simulink model "HANcoder_E407_SMV_program"  (R2018a)
settings: Solver=FixedStepDiscrete  StartTime=0.0  StopTime=1  FixedStep=0.01  RelTol=1e-3
PreLoadFcn:
  | librarySetup
  | eval([bdroot,'_startup']) %Calling [modelName]_startup.m
values from neighbouring files (symbols this model uses):
  Speed = [0.4; 0.4; 0.4; 0.4; 0.4; 0.4; 0.4; 0.4; 0.4; 0.4;0]    [Xbee_Track_Presentation.m]
undefined symbols (not defined in the file or in its folder): A0, A1, A2, A3, b, CON2, CON3, CON4, D13, D4, D5, drivemode, L_D1, L_D2, manual_xbee_switch, Steering_angle, steermode
libraries: HANcoder_STM32_Target x38, simulink_extras x11, simulink x7
(part 2 of 3)

== system HANcoder_E407_SMV_program/HANcoder STM32 Target - E407-STM32 algorithm/Xbee controll/Error value als het nodig is ==
  ThrottleIn : Inport
  SteeringIn : Inport  Port=2
  SteeringOut : Outport
  ThrottleOut : Outport  Port=2
  wires:
  ThrottleIn/1 -> ThrottleOut/1
  SteeringIn/1 -> SteeringOut/1

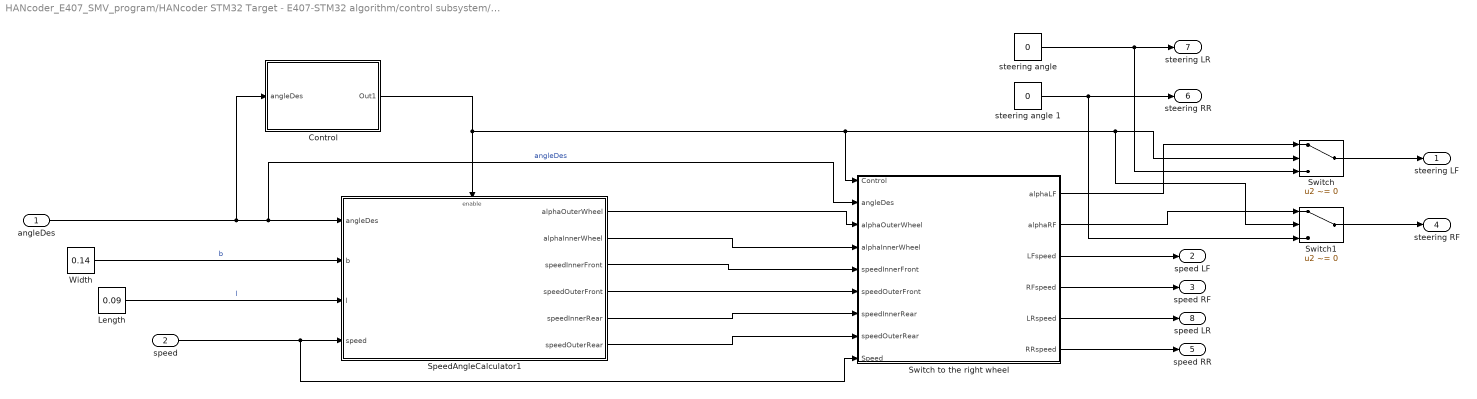
== system HANcoder_E407_SMV_program/HANcoder STM32 Target - E407-STM32 algorithm/control subsystem/2 wheel steering ==
  angleDes : Inport
  speed : Inport  Port=2
  Control : Subsystem
  Length : Constant  Value=0.09
  SpeedAngleCalculator1 : Subsystem
  Switch : Switch  Criteria=u2 ~= 0
  "Switch to the right wheel " : Subsystem
  Switch1 : Switch  Criteria=u2 ~= 0
  Width : Constant  Value=0.14
  "steering angle " : Constant  Value=0
  steering angle 1 : Constant  Value=0
  steering LF : Outport
  speed LF : Outport  Port=2
  speed RF : Outport  Port=3
  steering RF : Outport  Port=4
  speed RR : Outport  Port=5
  steering RR : Outport  Port=6
  steering LR : Outport  Port=7
  speed LR : Outport  Port=8
  wires:
  "steering angle "/1 -> Switch/3, steering LR/1
  steering angle 1/1 -> Switch1/3, steering RR/1
  "Switch to the right wheel "/4(RFspeed) -> speed RF/1
  angleDes/1 -> Control/1(angleDes), "Switch to the right wheel "/2(angleDes), SpeedAngleCalculator1/1(angleDes)  "angleDes"
  "Switch to the right wheel "/5(LRspeed) -> speed LR/1
  "Switch to the right wheel "/6(RRspeed) -> speed RR/1
  speed/1 -> "Switch to the right wheel "/9(Speed), SpeedAngleCalculator1/4(speed)
  Width/1 -> SpeedAngleCalculator1/2(b)  "b"
  SpeedAngleCalculator1/2(alphaInnerWheel) -> "Switch to the right wheel "/4(alphaInnerWheel)
  SpeedAngleCalculator1/6(speedOuterRear) -> "Switch to the right wheel "/8(speedOuterRear)
  SpeedAngleCalculator1/5(speedInnerRear) -> "Switch to the right wheel "/7(speedInnerRear)
  Length/1 -> SpeedAngleCalculator1/3(l)  "l"
  SpeedAngleCalculator1/1(alphaOuterWheel) -> "Switch to the right wheel "/3(alphaOuterWheel)
  SpeedAngleCalculator1/3(speedInnerFront) -> "Switch to the right wheel "/5(speedInnerFront)
  "Switch to the right wheel "/3(LFspeed) -> speed LF/1
  SpeedAngleCalculator1/4(speedOuterFront) -> "Switch to the right wheel "/6(speedOuterFront)
  "Switch to the right wheel "/1(alphaLF) -> Switch/1
  Switch/1 -> steering LF/1
  Switch1/1 -> steering RF/1
  "Switch to the right wheel "/2(alphaRF) -> Switch1/1
  Control/1(Out1) -> "Switch to the right wheel "/1(Control), Switch1/2, Switch/2, SpeedAngleCalculator1/Enable

== system HANcoder_E407_SMV_program/HANcoder STM32 Target - E407-STM32 algorithm/control subsystem/4 wheel steering ==
  angleDes : Inport
  speed : Inport  Port=2
  Control : Subsystem
  Subsystem1 : Subsystem
  Switch to the right wheel (Don't open if you're smart)1 : Subsystem
  angleDes1 : InportShadow
  angleDes2 : InportShadow
  b : Constant  Value=0.14
  l : Constant  Value=0.09
  speed2 : InportShadow  Port=2
  steering LF : Outport
  speed LF : Outport  Port=2
  speed RF : Outport  Port=3
  steering RF : Outport  Port=4
  speed RR : Outport  Port=5
  steering RR : Outport  Port=6
  steering LR : Outport  Port=7
  speed LR : Outport  Port=8
  wires:
  Switch to the right wheel (Don't open if you're smart)1/5(LFspeed) -> speed LF/1
  Switch to the right wheel (Don't open if you're smart)1/4(steeringRR) -> steering RR/1
  Switch to the right wheel (Don't open if you're smart)1/8(RRspeed) -> speed RR/1
  Switch to the right wheel (Don't open if you're smart)1/3(steeringRF) -> steering RF/1
  Switch to the right wheel (Don't open if you're smart)1/2("steeringLR ") -> steering LR/1
  Switch to the right wheel (Don't open if you're smart)1/6(RFspeed) -> speed RF/1
  Switch to the right wheel (Don't open if you're smart)1/7(LRspeed) -> speed LR/1
  Switch to the right wheel (Don't open if you're smart)1/1(steeringLF) -> steering LF/1
  angleDes2/1 -> Switch to the right wheel (Don't open if you're smart)1/6(angleDes)
  speed/1 -> Switch to the right wheel (Don't open if you're smart)1/7(Speed)
  b/1 -> Subsystem1/3(b)
  Subsystem1/2(speedOuter) -> Switch to the right wheel (Don't open if you're smart)1/3(speedOuterFront)
  l/1 -> Subsystem1/1(l)
  Subsystem1/4(AlphaInner) -> Switch to the right wheel (Don't open if you're smart)1/5(alphaOuterWheel)
  Control/1(Control) -> Subsystem1/Enable, Switch to the right wheel (Don't open if you're smart)1/1(Control)
  Subsystem1/3(AlphaOuter) -> Switch to the right wheel (Don't open if you're smart)1/4(alphaInnerWheel)
  Subsystem1/1(speedInner) -> Switch to the right wheel (Don't open if you're smart)1/2(speedInnerFront)
  angleDes/1 -> Subsystem1/2(angleDes)
  angleDes1/1 -> Control/1(angleDes)
  speed2/1 -> Subsystem1/4(speed)

== system HANcoder_E407_SMV_program/HANcoder STM32 Target - E407-STM32 algorithm/control subsystem/axle enable ==
  Xbeedriveline : Inport
  incomingF : Inport  Port=2
  incomingR : Inport  Port=3
  Subsystem : Subsystem
  Subsystem1 : Subsystem
  Out1 : Outport
  Out2 : Outport  Port=2
  wires:
  Subsystem/1(zero1) -> Out2/1
  Subsystem1/1(zero) -> Out1/1
  Xbeedriveline/1 -> Subsystem/2(xbeedriveline), Subsystem1/2(xbeedriveline)
  incomingF/1 -> Subsystem1/1(incomingF)
  incomingR/1 -> Subsystem/1(incomingR)

== system HANcoder_E407_SMV_program/HANcoder STM32 Target - E407-STM32 algorithm/control subsystem/direction subsystem ==
  Xbeedrive : Inport
  Constant : Constant  Value=3
  Digital Output1 : HANcoder_STM32_Target/STM32-E407/Digital Outputs/Digital Output  Tag=HANcoder_TARGET_STM32_E407  pinID=CON PE - 4  config=Push pull  tsamp=-1
      settings: SourceProductName=HANcoder STM32 Target
  Sum : Sum  Inputs=|+-
  Switch : Switch  Threshold=4  OutDataTypeStr=boolean
  Switch1 : Switch  Threshold=1
  negDirection : Constant
  posDirection : Constant  Value=0
  Out1 : Outport
  wires:
  negDirection/1 -> Switch/1
  Xbeedrive/1 -> Switch1/3, Sum/1, Switch/2
  Switch/1 -> Switch1/2, Digital Output1/1  "direction"
  posDirection/1 -> Switch/3
  Constant/1 -> Sum/2
  Switch1/1 -> Out1/1
  Sum/1 -> Switch1/1

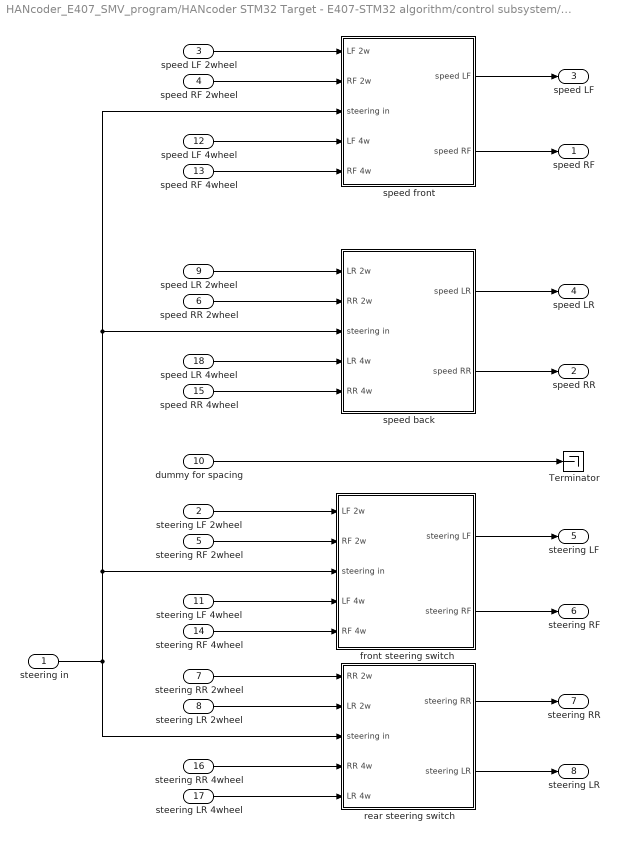
== system HANcoder_E407_SMV_program/HANcoder STM32 Target - E407-STM32 algorithm/control subsystem/steering switch ==
  steering in : Inport
  steering LF 2wheel : Inport  Port=2
  speed LF 2wheel : Inport  Port=3
  speed RF 2wheel : Inport  Port=4
  steering RF 2wheel : Inport  Port=5
  speed RR 2wheel : Inport  Port=6
  steering RR 2wheel : Inport  Port=7
  steering LR 2wheel : Inport  Port=8
  speed LR 2wheel : Inport  Port=9
  dummy for spacing : Inport  Port=10
  steering LF 4wheel : Inport  Port=11
  speed LF 4wheel : Inport  Port=12
  speed RF 4wheel : Inport  Port=13
  steering RF 4wheel : Inport  Port=14
  speed RR 4wheel : Inport  Port=15
  steering RR 4wheel : Inport  Port=16
  steering LR 4wheel : Inport  Port=17
  speed LR 4wheel : Inport  Port=18
  Terminator : Terminator
  front steering switch : Subsystem
  rear steering switch : Subsystem
  speed back : Subsystem
  speed front : Subsystem
  speed RF : Outport
  speed RR : Outport  Port=2
  speed LF : Outport  Port=3
  speed LR : Outport  Port=4
  steering LF : Outport  Port=5
  steering RF : Outport  Port=6
  steering RR : Outport  Port=7
  steering LR : Outport  Port=8
  wires:
  rear steering switch/1(steering RR) -> steering RR/1
  rear steering switch/2(steering LR) -> steering LR/1
  steering in/1 -> rear steering switch/3(steering in), speed front/3(steering in), speed back/3(steering in), front steering switch/3(steering in)
  speed LR 2wheel/1 -> speed back/1(LR 2w)
  speed LF 2wheel/1 -> speed front/1(LF 2w)
  speed LR 4wheel/1 -> speed back/4(LR 4w)
  speed RR 4wheel/1 -> speed back/5(RR 4w)
  speed RF 2wheel/1 -> speed front/2(RF 2w)
  speed RR 2wheel/1 -> speed back/2(RR 2w)
  front steering switch/2(steering RF) -> steering RF/1
  front steering switch/1(steering LF) -> steering LF/1
  speed LF 4wheel/1 -> speed front/4(LF 4w)
  speed RF 4wheel/1 -> speed front/5(RF 4w)
  steering LF 2wheel/1 -> front steering switch/1(LF 2w)
  steering RF 2wheel/1 -> front steering switch/2(RF 2w)
  steering LF 4wheel/1 -> front steering switch/4(LF 4w)
  steering RF 4wheel/1 -> front steering switch/5(RF 4w)
  steering RR 2wheel/1 -> rear steering switch/1(RR 2w)
  steering LR 2wheel/1 -> rear steering switch/2(LR 2w)
  steering RR 4wheel/1 -> rear steering switch/4(RR 4w)
  steering LR 4wheel/1 -> rear steering switch/5(LR 4w)
  speed front/1(speed LF) -> speed LF/1
  speed front/2(speed RF) -> speed RF/1
  speed back/1(speed LR) -> speed LR/1
  speed back/2(speed RR) -> speed RR/1
  dummy for spacing/1 -> Terminator/1

== system HANcoder_E407_SMV_program/HANcoder STM32 Target - E407-STM32 algorithm/initialisation/Output Compare Init1 ==
  S-Function : S-Function  FunctionName=sfcn_timeout_init  SFunctionDeploymentMode=off  EnableBusSupport=off
  Term1 : Terminator
  wires:
  S-Function/1 -> Term1/1

== system HANcoder_E407_SMV_program/HANcoder STM32 Target - E407-STM32 algorithm/initialisation/PWM Init ==
  S-Function : S-Function  FunctionName=sfcn_pwmout_init  SFunctionDeploymentMode=off  EnableBusSupport=off
  Term1 : Terminator
  wires:
  S-Function/1 -> Term1/1

== system HANcoder_E407_SMV_program/HANcoder STM32 Target - E407-STM32 algorithm/initialisation/PWM Init1 ==
  S-Function : S-Function  FunctionName=sfcn_pwmout_init  SFunctionDeploymentMode=off  EnableBusSupport=off
  Term1 : Terminator
  wires:
  S-Function/1 -> Term1/1

== system HANcoder_E407_SMV_program/HANcoder STM32 Target - E407-STM32 algorithm/initialisation/PWM Init2 ==
  S-Function : S-Function  FunctionName=sfcn_pwmout_init  SFunctionDeploymentMode=off  EnableBusSupport=off
  Term1 : Terminator
  wires:
  S-Function/1 -> Term1/1

== system HANcoder_E407_SMV_program/HANcoder STM32 Target - E407-STM32 algorithm/initialisation/UART init ==
  Level-2 M-file S-Function : M-S-Function  FunctionName=sfcn_uart_init
  Term1 : Terminator
  wires:
  Level-2 M-file S-Function/1 -> Term1/1

== system HANcoder_E407_SMV_program/HANcoder STM32 Target - E407-STM32 algorithm/output compare Left front/Subsystem2 ==
  In1 : Inport
  function : TriggerPort  TriggerType=function-call  VariantControl=(inherit)
  " 2: invert logic state of the outpin pin." : Constant  Value=2  OutDataTypeStr=uint8
  Gain : Gain  Commented=on  Gain=2  OutDataTypeStr=uint16
  Get Free Running Counter1 : HANcoder_STM32_Target/STM32-E407/Timer Outputs/Get Free Running Counter  Tag=HANcoder_TARGET_STM32_E407  moduleID=TIM1 - CON PE - 12 & 14 & 16 & 17  tsamp=-1
      settings: SourceProductName=HANcoder STM32 Target
  Schedule Compare Event1 : HANcoder_STM32_Target/STM32-E407/Timer Outputs/Schedule Compare Event  Tag=HANcoder_TARGET_STM32_E407  pin=TIM1 - CON PE - 12 - 5V Tolerant  tsamp=-1
      settings: SourceProductName=HANcoder STM32 Target
  Sum : Sum  Inputs=|++
  wires:
  " 2: invert logic state of the outpin pin."/1 -> Schedule Compare Event1/2
  Get Free Running Counter1/1 -> Sum/2
  Sum/1 -> Schedule Compare Event1/1
  In1/1 -> Sum/1

== system HANcoder_E407_SMV_program/HANcoder STM32 Target - E407-STM32 algorithm/output compare Left front/calculated frequency ==
  ticks : Inport
  Constant : Constant  Value=10000000  OutDataTypeStr=uint32
  Divide : Product  Inputs=*/  OutDataTypeStr=uint32
  Gain : Gain  Gain=2  OutDataTypeStr=uint16
  Product : Product
  Terminator : Terminator
  t_tick times 10^7 : Constant  Value=5  OutDataTypeStr=uint8
  wires:
  Constant/1 -> Divide/1
  Product/1 -> Divide/2
  Gain/1 -> Product/1
  t_tick times 10^7/1 -> Product/2
  Divide/1 -> Terminator/1  "freq_calc_LF"
  ticks/1 -> Gain/1

== system HANcoder_E407_SMV_program/HANcoder STM32 Target - E407-STM32 algorithm/output compare Left front/ms to tick conversion ==
  note: rad/s
  m/s : Inport
  Constant2 : Constant
  Divide1 : Product  Inputs=*/  OutDataTypeStr=uint16
  Gain : Gain  Gain=2
  Gain1 : Gain  Gain=0.0000005
  Gain2 : Gain  Gain=2*pi
  Gain3 : Gain  Gain=200
  wheel radius : Gain  Gain=1/0.0405
  Out1 : Outport
  wires:
  Constant2/1 -> Gain2/1
  Gain/1 -> Gain1/1
  m/s/1 -> wheel radius/1
  Gain1/1 -> Gain3/1
  Divide1/1 -> Out1/1
  Gain2/1 -> Divide1/1
  Gain3/1 -> Divide1/2
  wheel radius/1 -> Gain/1

== system HANcoder_E407_SMV_program/HANcoder STM32 Target - E407-STM32 algorithm/output compare Left front/start scheduling for output compare ==
  Trigger : TriggerPort  TriggerType=either  VariantControl=(inherit)  InitialTriggerSignalState=zero  PortDimensions=1
  "  3: do nothing to the output pin." : Constant  Value=3  OutDataTypeStr=uint8
  Schedule Compare Event : HANcoder_STM32_Target/STM32-E407/Timer Outputs/Schedule Compare Event  Tag=HANcoder_TARGET_STM32_E407  pin=TIM1 - CON PE - 12 - 5V Tolerant  tsamp=-1
      settings: SourceProductName=HANcoder STM32 Target
  zero value : Constant  Value=0  OutDataTypeStr=uint16
  wires:
  "  3: do nothing to the output pin."/1 -> Schedule Compare Event/2
  zero value/1 -> Schedule Compare Event/1

== system HANcoder_E407_SMV_program/HANcoder STM32 Target - E407-STM32 algorithm/output compare left rear/Subsystem2 ==
  In1 : Inport
  function : TriggerPort  TriggerType=function-call  VariantControl=(inherit)
  " 2: invert logic state of the outpin pin." : Constant  Value=2  OutDataTypeStr=uint8
  Get Free Running Counter1 : HANcoder_STM32_Target/STM32-E407/Timer Outputs/Get Free Running Counter  Tag=HANcoder_TARGET_STM32_E407  moduleID=TIM1 - CON PE - 12 & 14 & 16 & 17  tsamp=-1
      settings: SourceProductName=HANcoder STM32 Target
  Schedule Compare Event1 : HANcoder_STM32_Target/STM32-E407/Timer Outputs/Schedule Compare Event  Tag=HANcoder_TARGET_STM32_E407  pin=TIM1 - CON PE - 17 - 5V Tolerant  tsamp=-1
      settings: SourceProductName=HANcoder STM32 Target
  Sum : Sum  Inputs=|++  OutDataTypeStr=uint16
  wires:
  Sum/1 -> Schedule Compare Event1/1
  Get Free Running Counter1/1 -> Sum/2
  " 2: invert logic state of the outpin pin."/1 -> Schedule Compare Event1/2
  In1/1 -> Sum/1

== system HANcoder_E407_SMV_program/HANcoder STM32 Target - E407-STM32 algorithm/output compare left rear/Subsystem3 ==
  Trigger : TriggerPort  TriggerType=either  VariantControl=(inherit)  InitialTriggerSignalState=zero  PortDimensions=1
  "  3: do nothing to the output pin." : Constant  Value=3  OutDataTypeStr=uint8
  Schedule Compare Event1 : HANcoder_STM32_Target/STM32-E407/Timer Outputs/Schedule Compare Event  Tag=HANcoder_TARGET_STM32_E407  pin=TIM1 - CON PE - 16 - 5V Tolerant  tsamp=-1
      settings: SourceProductName=HANcoder STM32 Target
  zero value : Constant  Value=0  OutDataTypeStr=uint16
  wires:
  zero value/1 -> Schedule Compare Event1/1
  "  3: do nothing to the output pin."/1 -> Schedule Compare Event1/2

== system HANcoder_E407_SMV_program/HANcoder STM32 Target - E407-STM32 algorithm/output compare left rear/calculated frequency ==
  ticks : Inport
  Constant : Constant  Value=10000000  OutDataTypeStr=uint32
  Divide : Product  Inputs=*/  OutDataTypeStr=uint32
  Gain : Gain  Gain=2  OutDataTypeStr=uint16
  Product : Product
  Terminator : Terminator
  t_tick times 10^7 : Constant  Value=5  OutDataTypeStr=uint8
  wires:
  Constant/1 -> Divide/1
  Product/1 -> Divide/2
  Gain/1 -> Product/1
  t_tick times 10^7/1 -> Product/2
  Divide/1 -> Terminator/1
  ticks/1 -> Gain/1

== system HANcoder_E407_SMV_program/HANcoder STM32 Target - E407-STM32 algorithm/output compare left rear/rad to tick conversion ==
  In1 : Inport
  Constant2 : Constant
  Divide1 : Product  Inputs=*/  OutDataTypeStr=uint16
  Gain : Gain  Gain=2
  Gain1 : Gain  Gain=0.0000005
  Gain2 : Gain  Gain=2*pi
  Gain3 : Gain  Gain=200
  wheel radius : Gain  Gain=1/0.0405
  Out1 : Outport
  wires:
  Constant2/1 -> Gain2/1
  Gain/1 -> Gain1/1
  In1/1 -> wheel radius/1
  Gain1/1 -> Gain3/1
  Divide1/1 -> Out1/1
  Gain2/1 -> Divide1/1
  Gain3/1 -> Divide1/2
  wheel radius/1 -> Gain/1

== system HANcoder_E407_SMV_program/HANcoder STM32 Target - E407-STM32 algorithm/output compare right front/Subsystem2 ==
  In1 : Inport
  function : TriggerPort  TriggerType=function-call  VariantControl=(inherit)
  " 2: invert logic state of the outpin pin." : Constant  Value=2  OutDataTypeStr=uint8
  Gain : Gain  Commented=on  Gain=2  OutDataTypeStr=uint16
  Get Free Running Counter1 : HANcoder_STM32_Target/STM32-E407/Timer Outputs/Get Free Running Counter  Tag=HANcoder_TARGET_STM32_E407  moduleID=TIM1 - CON PE - 12 & 14 & 16 & 17  tsamp=-1
      settings: SourceProductName=HANcoder STM32 Target
  Schedule Compare Event1 : HANcoder_STM32_Target/STM32-E407/Timer Outputs/Schedule Compare Event  Tag=HANcoder_TARGET_STM32_E407  pin=TIM1 - CON PE - 14 - 5V Tolerant  tsamp=-1
      settings: SourceProductName=HANcoder STM32 Target
  Sum : Sum  Inputs=|++
  wires:
  Sum/1 -> Schedule Compare Event1/1  "event_counter_RF"
  Get Free Running Counter1/1 -> Sum/2  "FRC_value_RF"
  " 2: invert logic state of the outpin pin."/1 -> Schedule Compare Event1/2
  In1/1 -> Sum/1

== system HANcoder_E407_SMV_program/HANcoder STM32 Target - E407-STM32 algorithm/output compare right front/Subsystem3 ==
  Trigger : TriggerPort  TriggerType=either  VariantControl=(inherit)  InitialTriggerSignalState=zero  PortDimensions=1
  "  3: do nothing to the output pin." : Constant  Value=3  OutDataTypeStr=uint8
  Schedule Compare Event1 : HANcoder_STM32_Target/STM32-E407/Timer Outputs/Schedule Compare Event  Tag=HANcoder_TARGET_STM32_E407  pin=TIM1 - CON PE - 14 - 5V Tolerant  tsamp=-1
      settings: SourceProductName=HANcoder STM32 Target
  zero value : Constant  Value=0  OutDataTypeStr=uint16
  wires:
  zero value/1 -> Schedule Compare Event1/1
  "  3: do nothing to the output pin."/1 -> Schedule Compare Event1/2

== system HANcoder_E407_SMV_program/HANcoder STM32 Target - E407-STM32 algorithm/output compare right front/calculated frequency ==
  ticks : Inport
  Constant : Constant  Value=10000000  OutDataTypeStr=uint32
  Divide : Product  Inputs=*/  OutDataTypeStr=uint32
  Gain : Gain  Gain=2  OutDataTypeStr=uint16
  Product : Product
  Terminator : Terminator
  t_tick times 10^7 : Constant  Value=5  OutDataTypeStr=uint8
  wires:
  Constant/1 -> Divide/1
  Product/1 -> Divide/2
  Gain/1 -> Product/1
  t_tick times 10^7/1 -> Product/2
  Divide/1 -> Terminator/1
  ticks/1 -> Gain/1

== system HANcoder_E407_SMV_program/HANcoder STM32 Target - E407-STM32 algorithm/output compare right front/rad to tick conversion ==
  In1 : Inport
  Constant2 : Constant
  Divide1 : Product  Inputs=*/  OutDataTypeStr=uint16
  Gain : Gain  Gain=2
  Gain1 : Gain  Gain=0.0000005
  Gain2 : Gain  Gain=2*pi
  Gain3 : Gain  Gain=200
  wheel radius : Gain  Gain=1/0.0405
  Out1 : Outport
  wires:
  Constant2/1 -> Gain2/1
  Gain/1 -> Gain1/1
  In1/1 -> wheel radius/1
  Gain1/1 -> Gain3/1
  Divide1/1 -> Out1/1
  Gain2/1 -> Divide1/1
  Gain3/1 -> Divide1/2
  wheel radius/1 -> Gain/1

== system HANcoder_E407_SMV_program/HANcoder STM32 Target - E407-STM32 algorithm/output compare right rear/Subsystem2 ==
  In1 : Inport
  function : TriggerPort  TriggerType=function-call  VariantControl=(inherit)
  " 2: invert logic state of the outpin pin." : Constant  Value=2  OutDataTypeStr=uint8
  Get Free Running Counter1 : HANcoder_STM32_Target/STM32-E407/Timer Outputs/Get Free Running Counter  Tag=HANcoder_TARGET_STM32_E407  moduleID=TIM1 - CON PE - 12 & 14 & 16 & 17  tsamp=-1
      settings: SourceProductName=HANcoder STM32 Target
  Schedule Compare Event1 : HANcoder_STM32_Target/STM32-E407/Timer Outputs/Schedule Compare Event  Tag=HANcoder_TARGET_STM32_E407  pin=TIM1 - CON PE - 16 - 5V Tolerant  tsamp=-1
      settings: SourceProductName=HANcoder STM32 Target
  Sum : Sum  Inputs=|++
  wires:
  " 2: invert logic state of the outpin pin."/1 -> Schedule Compare Event1/2
  Get Free Running Counter1/1 -> Sum/2
  Sum/1 -> Schedule Compare Event1/1
  In1/1 -> Sum/1

== system HANcoder_E407_SMV_program/HANcoder STM32 Target - E407-STM32 algorithm/output compare right rear/Subsystem3 ==
  Trigger : TriggerPort  TriggerType=either  VariantControl=(inherit)  InitialTriggerSignalState=zero  PortDimensions=1
  "  3: do nothing to the output pin." : Constant  Value=3  OutDataTypeStr=uint8
  Schedule Compare Event1 : HANcoder_STM32_Target/STM32-E407/Timer Outputs/Schedule Compare Event  Tag=HANcoder_TARGET_STM32_E407  pin=TIM1 - CON PE - 17 - 5V Tolerant  tsamp=-1
      settings: SourceProductName=HANcoder STM32 Target
  zero value : Constant  Value=0  OutDataTypeStr=uint16
  wires:
  "  3: do nothing to the output pin."/1 -> Schedule Compare Event1/2
  zero value/1 -> Schedule Compare Event1/1

== system HANcoder_E407_SMV_program/HANcoder STM32 Target - E407-STM32 algorithm/output compare right rear/calculated frequency ==
  ticks : Inport
  Constant : Constant  Value=10000000  OutDataTypeStr=uint32
  Divide : Product  Inputs=*/  OutDataTypeStr=uint32
  Gain : Gain  Gain=2  OutDataTypeStr=uint16
  Product : Product
  Terminator : Terminator
  t_tick times 10^7 : Constant  Value=5  OutDataTypeStr=uint8
  wires:
  Constant/1 -> Divide/1
  Product/1 -> Divide/2
  Gain/1 -> Product/1
  t_tick times 10^7/1 -> Product/2
  Divide/1 -> Terminator/1
  ticks/1 -> Gain/1

== system HANcoder_E407_SMV_program/HANcoder STM32 Target - E407-STM32 algorithm/output compare right rear/ms to tick conversion ==
  note: m/s to rad/s conversion
  In1 : Inport
  Constant2 : Constant
  Divide1 : Product  Inputs=*/  OutDataTypeStr=uint16
  Gain : Gain  Gain=2
  Gain1 : Gain  Gain=0.0000005
  Gain2 : Gain  Gain=2*pi
  Gain3 : Gain  Gain=200
  wheel radius : Gain  Gain=1/0.0405
  Out1 : Outport
  wires:
  Constant2/1 -> Gain2/1
  Gain/1 -> Gain1/1
  In1/1 -> wheel radius/1
  Gain1/1 -> Gain3/1
  Divide1/1 -> Out1/1
  Gain2/1 -> Divide1/1
  Gain3/1 -> Divide1/2
  wheel radius/1 -> Gain/1

== system HANcoder_E407_SMV_program/HANcoder STM32 Target - E407-STM32 algorithm/Steering Drive Control/Subsystem3/If Action Subsystem ==
  Axle1_Left_steering [rad] : Inport
  Axle1_Right_steering [rad] : Inport  Port=2
  Action Port : ActionPort
  Constant : Constant  Value=0
  Constant1 : Constant  Value=0
  Axle1_Left_steering[rad] : Outport
  Axle1_Right_steering[rad] : Outport  Port=2
  Axle2_Left_steering[rad] : Outport  Port=3
  Axle2_Right_steering[rad] : Outport  Port=4
  wires:
  Axle1_Left_steering [rad]/1 -> Axle1_Left_steering[rad]/1
  Axle1_Right_steering [rad]/1 -> Axle1_Right_steering[rad]/1
  Constant/1 -> Axle2_Left_steering[rad]/1
  Constant1/1 -> Axle2_Right_steering[rad]/1

== system HANcoder_E407_SMV_program/HANcoder STM32 Target - E407-STM32 algorithm/Steering Drive Control/Subsystem3/If Action Subsystem1 ==
  Axle2_Left_steering [rad] : Inport
  Axle2_Right_steering [rad] : Inport  Port=2
  Action Port : ActionPort
  Constant : Constant  Value=0
  Constant1 : Constant  Value=0
  Axle1_Left_steering[rad] : Outport
  Axle1_Right_steering[rad] : Outport  Port=2
  Axle2_Left_steering[rad] : Outport  Port=3
  Axle2_Right_steering[rad] : Outport  Port=4
  wires:
  Axle2_Left_steering [rad]/1 -> Axle2_Left_steering[rad]/1
  Axle2_Right_steering [rad]/1 -> Axle2_Right_steering[rad]/1
  Constant/1 -> Axle1_Left_steering[rad]/1
  Constant1/1 -> Axle1_Right_steering[rad]/1

== system HANcoder_E407_SMV_program/HANcoder STM32 Target - E407-STM32 algorithm/Steering Drive Control/Subsystem3/If Action Subsystem2 ==
  Axle1_Left_steering [rad] : Inport
  Axle1_Right_steering [rad] : Inport  Port=2
  Axle2_Left_steering [rad] : Inport  Port=3
  Axle2_Right_steering [rad] : Inport  Port=4
  Action Port : ActionPort
  Axle1_Left_steering[rad] : Outport
  Axle1_Right_steering[rad] : Outport  Port=2
  Axle2_Left_steering[rad] : Outport  Port=3
  Axle2_Right_steering[rad] : Outport  Port=4
  wires:
  Axle1_Left_steering [rad]/1 -> Axle1_Left_steering[rad]/1
  Axle1_Right_steering [rad]/1 -> Axle1_Right_steering[rad]/1
  Axle2_Left_steering [rad]/1 -> Axle2_Left_steering[rad]/1
  Axle2_Right_steering [rad]/1 -> Axle2_Right_steering[rad]/1

== system HANcoder_E407_SMV_program/HANcoder STM32 Target - E407-STM32 algorithm/Steering Drive Control/Subsystem3/If Action Subsystem3 ==
  Action Port : ActionPort
  Zero{,1..3} (4 alike) : Constant  Value=0
  Axle1_Left_steering[rad] : Outport
  Axle1_Right_steering[rad] : Outport  Port=2
  Axle2_Left_steering[rad] : Outport  Port=3
  Axle2_Right_steering[rad] : Outport  Port=4
  wires:
  Zero3/1 -> Axle2_Right_steering[rad]/1
  Zero2/1 -> Axle2_Left_steering[rad]/1
  Zero1/1 -> Axle1_Right_steering[rad]/1
  Zero/1 -> Axle1_Left_steering[rad]/1

== system HANcoder_E407_SMV_program/HANcoder STM32 Target - E407-STM32 algorithm/Steering Drive Control/Subsystem4/If Action Subsystem ==
  In1 : Inport
  Action Port : ActionPort
  Out1 : Outport
  wires:
  In1/1 -> Out1/1

== system HANcoder_E407_SMV_program/HANcoder STM32 Target - E407-STM32 algorithm/System information/debug led/Algorithm ==
  note: The button or the HANtuneOverride parameter
      | switches between the two frequencies.
  note: Here the algorithm can be placed. No hardware dependent blocks should be used here.
  note: Switch LED frequency when button is pressed
  Button : Inport
  10Hz Counter Limiter : simulink/Sources/Counter Limited  uplimit=1  tsamp=0.1
  5Hz Counter Limited : simulink/Sources/Counter Limited  uplimit=1  tsamp=0.2
  Data Type Conversion : DataTypeConversion  OutDataTypeStr=boolean
  Switch : Switch  Criteria=u2 > Threshold
  LED : Outport
  wires:
  Data Type Conversion/1 -> LED/1  "LedValue"
  5Hz Counter Limited/1 -> Switch/3
  Switch/1 -> Data Type Conversion/1
  Button/1 -> Switch/2
  10Hz Counter Limiter/1 -> Switch/1

== system HANcoder_E407_SMV_program/HANcoder STM32 Target - E407-STM32 algorithm/System information/debug led/Inputs ==
  note: The inputs and outputs are kept in a separate subsystem, this way the algorithm can easily be transferred to different hardware
  Digital Input : HANcoder_STM32_Target/STM32-E407/Digital Inputs/Digital Input  Tag=HANcoder_TARGET_STM32_E407  pinID=WKUP button  config=Pulldown  tsamp=-1
      settings: SourceProductName=HANcoder STM32 Target
  Button : Outport
  wires:
  Digital Input/1 -> Button/1

== system HANcoder_E407_SMV_program/HANcoder STM32 Target - E407-STM32 algorithm/System information/debug led/Outputs ==
  note: The inputs and outputs are kept in a separate subsystem, this way the algorithm can easily be transferred to different hardware
  LED : Inport
  Digital Output : HANcoder_STM32_Target/STM32-E407/Digital Outputs/Digital Output  Tag=HANcoder_TARGET_STM32_E407  pinID=LED  config=Push pull  tsamp=-1
      settings: SourceProductName=HANcoder STM32 Target
  wires:
  LED/1 -> Digital Output/1

== system HANcoder_E407_SMV_program/HANcoder STM32 Target - E407-STM32 algorithm/Xbee controll/Check received data/Check next 3 bytes and send via CAN ==
  note: Only use the signals when the last byte is valid
  note: This should be replaced by a checksum
  note: Here we check the next three bytes, the priority determines which byte is read first from the buffer. Priority can be changed by right clicking the block and selecting properties
  Action Port : ActionPort
  Check if it is the stop byte : simulink/Logic and Bit Operations/Compare To Constant  relop===  const=253  OutDataTypeStr=uint8
  Enabled Subsystem : Subsystem  TreatAsAtomicUnit=on
  UART stop : Subsystem  Tag=HANcoder_TARGET_STM32_E407  Priority=30  AncestorBlock=HANcoder_STM32_Target/STM32-E407/UART/UART receive  mask(UART receive){channel=UART1: CON3 - D1 & D0, useStatusOut=off, tsamp=-1}
      mask prompts: useStatusOut "Use status outport"; tsamp "Sample time"
      mask help:
      | Function
      | ==========
      | Reads a byte from the UART reception buffer.
      |
      | Parameters per channel
      | ======================
      | - Select channel (TX & RX)
      | - Select if the status output should be enabled.
      |
      | Outputs
      | =======
      | - The value of the receive byte.
      | - When the status output is 0, the reception buffer was empty.
      mask init:
      | uartChannelInfoStr = sfcn_uart_receive_mcb(2, channel, useStatusOut);
      settings: MoveFcn=drawLogos
      mask Help: web('sfcn_uart_receive.html')
      mask TypeOptions channel: UART1: CON3 - D1 & D0 | UART2: CON PD - 8 & 9 | UART3: CON PD - 11 & 12 | UART6: UEXT - 3 & 4
      mask Display: fprintf('UART receive\n%s', uartChannelInfoStr);patch([240 246 246],[8 14 2],[1 0 0]);patch([248 248 254],[14 2 8],[0 0 0.35]);
  UART value1 : Subsystem  Tag=HANcoder_TARGET_STM32_E407  Priority=10  AncestorBlock=HANcoder_STM32_Target/STM32-E407/UART/UART receive  mask(UART receive){channel=UART1: CON3 - D1 & D0, useStatusOut=off, tsamp=-1}
      mask prompts: useStatusOut "Use status outport"; tsamp "Sample time"
      mask help:
      | Function
      | ==========
      | Reads a byte from the UART reception buffer.
      |
      | Parameters per channel
      | ======================
      | - Select channel (TX & RX)
      | - Select if the status output should be enabled.
      |
      | Outputs
      | =======
      | - The value of the receive byte.
      | - When the status output is 0, the reception buffer was empty.
      mask init:
      | uartChannelInfoStr = sfcn_uart_receive_mcb(2, channel, useStatusOut);
      settings: MoveFcn=drawLogos
      mask Help: web('sfcn_uart_receive.html')
      mask TypeOptions channel: UART1: CON3 - D1 & D0 | UART2: CON PD - 8 & 9 | UART3: CON PD - 11 & 12 | UART6: UEXT - 3 & 4
      mask Display: fprintf('UART receive\n%s', uartChannelInfoStr);patch([240 246 246],[8 14 2],[1 0 0]);patch([248 248 254],[14 2 8],[0 0 0.35]);
  UART value2 : Subsystem  Tag=HANcoder_TARGET_STM32_E407  Priority=20  AncestorBlock=HANcoder_STM32_Target/STM32-E407/UART/UART receive  mask(UART receive){channel=UART1: CON3 - D1 & D0, useStatusOut=off, tsamp=-1}
      mask prompts: useStatusOut "Use status outport"; tsamp "Sample time"
      mask help:
      | Function
      | ==========
      | Reads a byte from the UART reception buffer.
      |
      | Parameters per channel
      | ======================
      | - Select channel (TX & RX)
      | - Select if the status output should be enabled.
      |
      | Outputs
      | =======
      | - The value of the receive byte.
      | - When the status output is 0, the reception buffer was empty.
      mask init:
      | uartChannelInfoStr = sfcn_uart_receive_mcb(2, channel, useStatusOut);
      settings: MoveFcn=drawLogos
      mask Help: web('sfcn_uart_receive.html')
      mask TypeOptions channel: UART1: CON3 - D1 & D0 | UART2: CON PD - 8 & 9 | UART3: CON PD - 11 & 12 | UART6: UEXT - 3 & 4
      mask Display: fprintf('UART receive\n%s', uartChannelInfoStr);patch([240 246 246],[8 14 2],[1 0 0]);patch([248 248 254],[14 2 8],[0 0 0.35]);
  Throttle : Outport
  Steering : Outport  Port=2
  wires:
  UART stop/1(Out1) -> Check if it is the stop byte/1
  Check if it is the stop byte/1 -> Enabled Subsystem/Enable
  UART value1/1(Out1) -> Enabled Subsystem/1(In1)
  UART value2/1(Out1) -> Enabled Subsystem/2(In2)
  Enabled Subsystem/1(Out1) -> Throttle/1
  Enabled Subsystem/2(Out2) -> Steering/1

== system HANcoder_E407_SMV_program/HANcoder STM32 Target - E407-STM32 algorithm/Xbee controll/Check received data/Check received data ==
  note: Here we check if the start byte is the first byte in the buffer, if not it will read 1 byte and thus deleting this one from the buffer
  Action Port : ActionPort
  Check next 3 bytes and send via CAN : Subsystem  TreatAsAtomicUnit=on
  Constant : Constant
  drive_mode : Outport
  steer_mode : Outport  Port=2
  wires:
  Check next 3 bytes and send via CAN/1(drive_mode) -> drive_mode/1
  Check next 3 bytes and send via CAN/2(steer_mode) -> steer_mode/1
  Constant/1 -> Check next 3 bytes and send via CAN/Enable

== system HANcoder_E407_SMV_program/HANcoder STM32 Target - E407-STM32 algorithm/Xbee controll/Check received data/UART start ==
  Level-2 M-file S-Function : M-S-Function  FunctionName=sfcn_uart_receive  Parameters=tsamp
  Term1 : Terminator
  Out1 : Outport
  wires:
  Level-2 M-file S-Function/2 -> Term1/1
  Level-2 M-file S-Function/1 -> Out1/1

== system HANcoder_E407_SMV_program/HANcoder STM32 Target - E407-STM32 algorithm/control subsystem/2 wheel steering/Control ==
  angleDes : Inport
  ControlValue : Constant  Value=0
  Logical Operator : Logic  Operator=OR  AllPortsSameDT=off  OutDataTypeStr=boolean
  Out1 : Outport
  wires:
  angleDes/1 -> Logical Operator/2
  Logical Operator/1 -> Out1/1
  ControlValue/1 -> Logical Operator/1

== system HANcoder_E407_SMV_program/HANcoder STM32 Target - E407-STM32 algorithm/control subsystem/2 wheel steering/SpeedAngleCalculator1 ==
  angleDes : Inport
  b : Inport  Port=2
  l : Inport  Port=3
  speed : Inport  Port=4
  Enable : EnablePort
  Speed calculator : Subsystem
  Steerangle calculator : Subsystem
  alphaOuterWheel : Outport
  alphaInnerWheel : Outport  Port=2
  speedInnerFront : Outport  Port=3
  speedOuterFront : Outport  Port=4
  speedInnerRear : Outport  Port=5
  speedOuterRear : Outport  Port=6
  wires:
  Speed calculator/3(speedInnerRear) -> speedInnerRear/1
  speed/1 -> Speed calculator/4(speedDes)  "speedDes"
  Speed calculator/4(speedOuter rear) -> speedOuterRear/1
  Steerangle calculator/5(radiusCoG) -> Speed calculator/5(radiusCoG)
  Steerangle calculator/4(radiusInnerRear) -> Speed calculator/2(radiusInnerRear)
  Steerangle calculator/3(radiusOuterRear) -> Speed calculator/1(radiusOuterRear)
  angleDes/1 -> Steerangle calculator/1(angleDes)
  l/1 -> Speed calculator/3(l), Steerangle calculator/2(l)
  b/1 -> Steerangle calculator/3(b)
  Steerangle calculator/1(alphaOuter) -> alphaOuterWheel/1
  Steerangle calculator/2(alphaInner) -> alphaInnerWheel/1
  Speed calculator/1(speedInnerFront) -> speedInnerFront/1
  Speed calculator/2(speedOuterFront) -> speedOuterFront/1

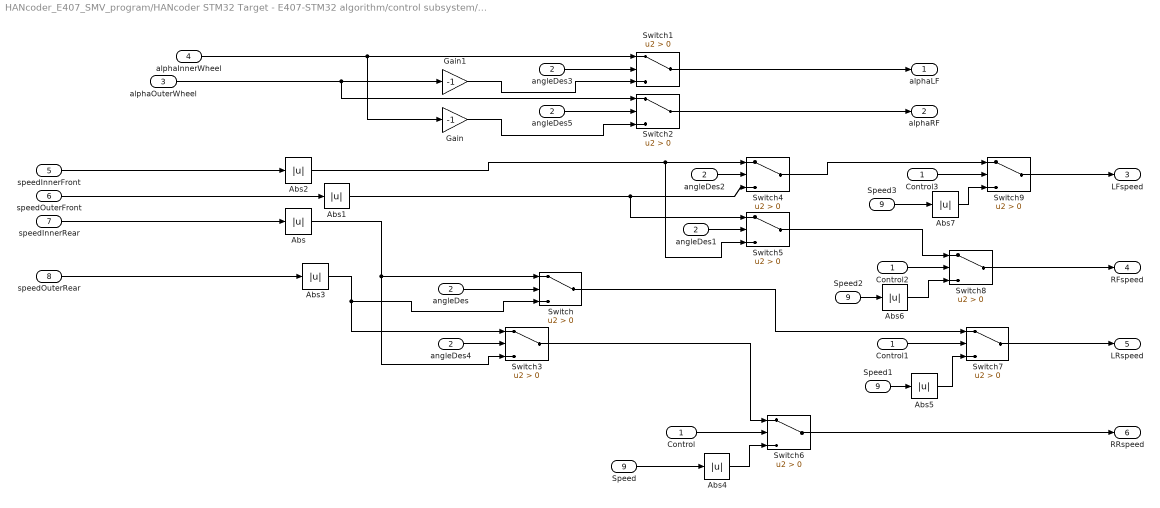
== system HANcoder_E407_SMV_program/HANcoder STM32 Target - E407-STM32 algorithm/control subsystem/2 wheel steering/Switch to the right wheel  ==
  Control : Inport
  angleDes : Inport  Port=2
  alphaOuterWheel : Inport  Port=3
  alphaInnerWheel : Inport  Port=4
  speedInnerFront : Inport  Port=5
  speedOuterFront : Inport  Port=6
  speedInnerRear : Inport  Port=7
  speedOuterRear : Inport  Port=8
  Speed : Inport  Port=9
  Abs{,1..7} (8 alike) : Abs
  Control1 : InportShadow
  Control2 : InportShadow
  Control3 : InportShadow
  Gain : Gain  Gain=-1
  Gain1 : Gain  Gain=-1
  Speed1 : InportShadow  Port=9
  Speed2 : InportShadow  Port=9
  Speed3 : InportShadow  Port=9
  Switch{,1..9} (10 alike) : Switch  Criteria=u2 > Threshold
  angleDes{1..5} (5 alike) : InportShadow  Port=2
  alphaLF : Outport
  alphaRF : Outport  Port=2
  LFspeed : Outport  Port=3
  RFspeed : Outport  Port=4
  LRspeed : Outport  Port=5
  RRspeed : Outport  Port=6
  wires:
  Abs2/1 -> Switch5/3, Switch4/1
  speedOuterFront/1 -> Abs1/1
  Switch1/1 -> alphaLF/1
  speedInnerRear/1 -> Abs/1
  speedInnerFront/1 -> Abs2/1
  Switch2/1 -> alphaRF/1
  Gain/1 -> Switch2/3
  speedOuterRear/1 -> Abs3/1
  Abs/1 -> Switch3/3, Switch/1
  Gain1/1 -> Switch1/3
  Abs1/1 -> Switch5/1, Switch4/3
  Abs3/1 -> Switch3/1, Switch/3
  angleDes3/1 -> Switch1/2
  angleDes2/1 -> Switch4/2
  angleDes1/1 -> Switch5/2
  angleDes/1 -> Switch/2
  angleDes4/1 -> Switch3/2
  angleDes5/1 -> Switch2/2
  Speed/1 -> Abs4/1
  Switch3/1 -> Switch6/1
  Switch6/1 -> RRspeed/1
  Control/1 -> Switch6/2
  Switch7/1 -> LRspeed/1
  Switch/1 -> Switch7/1
  Control1/1 -> Switch7/2
  Switch8/1 -> RFspeed/1
  Switch5/1 -> Switch8/1
  Speed2/1 -> Abs6/1
  Control2/1 -> Switch8/2
  Switch9/1 -> LFspeed/1
  Switch4/1 -> Switch9/1
  Control3/1 -> Switch9/2
  Speed3/1 -> Abs7/1
  Abs4/1 -> Switch6/3
  Abs5/1 -> Switch7/3
  Speed1/1 -> Abs5/1
  Abs6/1 -> Switch8/3
  Abs7/1 -> Switch9/3
  alphaOuterWheel/1 -> Switch2/1, Gain1/1
  alphaInnerWheel/1 -> Gain/1, Switch1/1

== system HANcoder_E407_SMV_program/HANcoder STM32 Target - E407-STM32 algorithm/control subsystem/4 wheel steering/Control ==
  angleDes : Inport
  ControlValue : Constant  Value=0
  Logical Operator : Logic  Operator=OR  AllPortsSameDT=off  OutDataTypeStr=boolean
  Control : Outport
  wires:
  Logical Operator/1 -> Control/1
  angleDes/1 -> Logical Operator/2
  ControlValue/1 -> Logical Operator/1

== system HANcoder_E407_SMV_program/HANcoder STM32 Target - E407-STM32 algorithm/control subsystem/4 wheel steering/Subsystem1 ==
  l : Inport
  angleDes : Inport  Port=2
  b : Inport  Port=3
  speed : Inport  Port=4
  Enable : EnablePort
  Angle inner wheels : Subsystem
  Angle outer wheels : Subsystem
  Angle to radius CoG : Subsystem
  radius inner wheel : Subsystem
  radius outer wheel : Subsystem
  speed calculator : Subsystem
  speedInner : Outport
  speedOuter : Outport  Port=2
  AlphaOuter : Outport  Port=3
  AlphaInner : Outport  Port=4
  wires:
  angleDes/1 -> Angle to radius CoG/2("angleDes ")
  Angle outer wheels/1(AlphaOuter) -> AlphaOuter/1
  l/1 -> radius inner wheel/1(l), radius outer wheel/1(l), Angle to radius CoG/1(l), Angle inner wheels/1(l), Angle outer wheels/1(l)
  b/1 -> radius inner wheel/2(b), radius outer wheel/2(b), Angle outer wheels/3(b), Angle inner wheels/3(b)
  speed calculator/1(speedInner) -> speedInner/1
  Angle to radius CoG/1(Rzw) -> Angle inner wheels/2(Rzw), radius outer wheel/3(Rzw), radius inner wheel/3(Rzw), Angle outer wheels/2(Rzw), speed calculator/2(Rzw)
  speed calculator/2(speedOuter) -> speedOuter/1
  Angle inner wheels/1(AlphaInner) -> AlphaInner/1
  radius inner wheel/1(radiusInner) -> speed calculator/3(radiusInner)
  radius outer wheel/1(radiusOuter) -> speed calculator/1(radiusOuter)
  speed/1 -> speed calculator/4(speed)

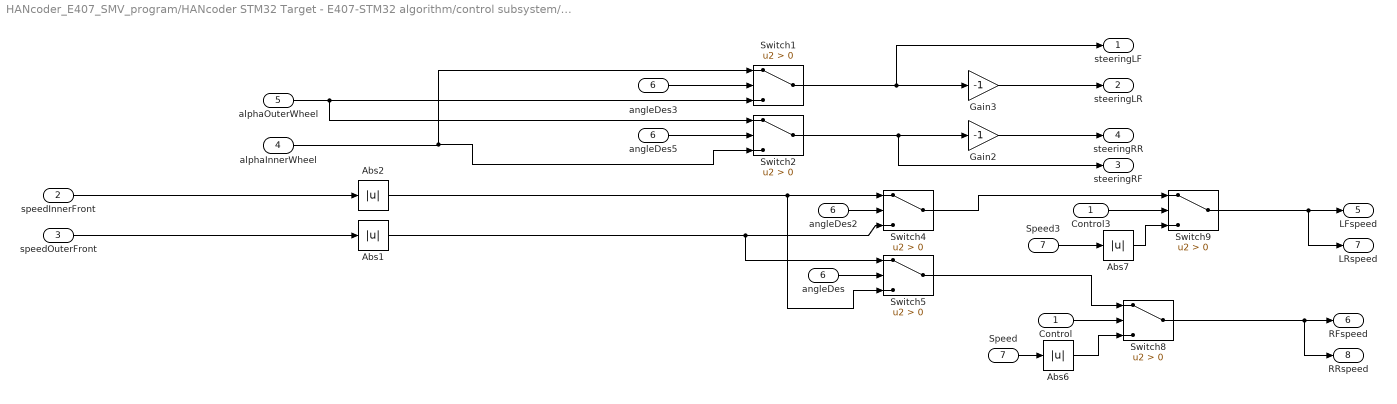
== system HANcoder_E407_SMV_program/HANcoder STM32 Target - E407-STM32 algorithm/control subsystem/4 wheel steering/Switch to the right wheel (Don't open if you're smart)1 ==
  Control : Inport
  speedInnerFront : Inport  Port=2
  speedOuterFront : Inport  Port=3
  alphaInnerWheel : Inport  Port=4
  alphaOuterWheel : Inport  Port=5
  angleDes : Inport  Port=6
  Speed : Inport  Port=7
  Abs{1..2,6..7} (4 alike) : Abs
  Control3 : InportShadow
  Gain2 : Gain  Gain=-1
  Gain3 : Gain  Gain=-1
  Speed3 : InportShadow  Port=7
  Switch{1..2,4..5,8..9} (6 alike) : Switch  Criteria=u2 > Threshold
  angleDes2 : InportShadow  Port=6
  angleDes3 : InportShadow  Port=6
  angleDes5 : InportShadow  Port=6
  steeringLF : Outport
  "steeringLR " : Outport  Port=2
  steeringRF : Outport  Port=3
  steeringRR : Outport  Port=4
  LFspeed : Outport  Port=5
  RFspeed : Outport  Port=6
  LRspeed : Outport  Port=7
  RRspeed : Outport  Port=8
  wires:
  Abs2/1 -> Switch5/3, Switch4/1
  speedOuterFront/1 -> Abs1/1
  speedInnerFront/1 -> Abs2/1
  alphaOuterWheel/1 -> Switch2/1, Switch1/3
  Abs1/1 -> Switch5/1, Switch4/3
  angleDes3/1 -> Switch1/2
  angleDes2/1 -> Switch4/2
  angleDes/1 -> Switch5/2
  angleDes5/1 -> Switch2/2
  Switch8/1 -> RRspeed/1, RFspeed/1
  Switch5/1 -> Switch8/1
  Speed/1 -> Abs6/1
  Control/1 -> Switch8/2
  Switch9/1 -> LRspeed/1, LFspeed/1
  Switch4/1 -> Switch9/1
  Control3/1 -> Switch9/2
  Speed3/1 -> Abs7/1
  Abs6/1 -> Switch8/3
  Abs7/1 -> Switch9/3
  Gain2/1 -> steeringRR/1
  Switch1/1 -> Gain3/1, steeringLF/1
  Switch2/1 -> steeringRF/1, Gain2/1
  Gain3/1 -> "steeringLR "/1
  alphaInnerWheel/1 -> Switch2/3, Switch1/1

== system HANcoder_E407_SMV_program/HANcoder STM32 Target - E407-STM32 algorithm/control subsystem/axle enable/Subsystem ==
  incomingR : Inport
  xbeedriveline : Inport  Port=2
  Compare To Constant : simulink/Logic and Bit Operations/Compare To Constant  relop=<=  const=1  OutDataTypeStr=boolean
  Constant2 : Constant  Value=0  OutDataTypeStr=boolean
  Constant3 : Constant  OutDataTypeStr=boolean
  Logical Operator : Logic  Operator=OR  AllPortsSameDT=off  OutDataTypeStr=boolean
  Switch1 : Switch  Criteria=u2 ~= 0
  zero1 : Outport
  wires:
  incomingR/1 -> Switch1/2
  Constant2/1 -> Switch1/1
  Switch1/1 -> Logical Operator/1
  Constant3/1 -> Switch1/3
  xbeedriveline/1 -> Compare To Constant/1
  Compare To Constant/1 -> Logical Operator/2
  Logical Operator/1 -> zero1/1

== system HANcoder_E407_SMV_program/HANcoder STM32 Target - E407-STM32 algorithm/control subsystem/axle enable/Subsystem1 ==
  incomingF : Inport
  xbeedriveline : Inport  Port=2
  Compare To Constant : simulink/Logic and Bit Operations/Compare To Constant  relop===  const=3  OutDataTypeStr=boolean
  Constant : Constant  Value=0  OutDataTypeStr=boolean
  Constant1 : Constant  OutDataTypeStr=boolean
  Logical Operator : Logic  Operator=OR  AllPortsSameDT=off  OutDataTypeStr=boolean
  Switch2 : Switch  Criteria=u2 ~= 0
  zero : Outport
  wires:
  incomingF/1 -> Switch2/2
  Constant/1 -> Switch2/1
  Constant1/1 -> Switch2/3
  Switch2/1 -> Logical Operator/1
  xbeedriveline/1 -> Compare To Constant/1
  Compare To Constant/1 -> Logical Operator/2
  Logical Operator/1 -> zero/1

== system HANcoder_E407_SMV_program/HANcoder STM32 Target - E407-STM32 algorithm/control subsystem/steering switch/front steering switch ==
  LF 2w : Inport
  RF 2w : Inport  Port=2
  steering in : Inport  Port=3
  LF 4w : Inport  Port=4
  RF 4w : Inport  Port=5
  Switch : Switch  Criteria=u2 > Threshold  Threshold=1
  Switch1 : Switch  Criteria=u2 > Threshold  Threshold=1
  steering in1 : InportShadow  Port=3
  steering LF : Outport
  steering RF : Outport  Port=2
  wires:
  LF 4w/1 -> Switch/1
  steering in1/1 -> Switch1/2
  Switch1/1 -> steering RF/1
  RF 2w/1 -> Switch1/3
  Switch/1 -> steering LF/1
  steering in/1 -> Switch/2
  RF 4w/1 -> Switch1/1
  LF 2w/1 -> Switch/3

== system HANcoder_E407_SMV_program/HANcoder STM32 Target - E407-STM32 algorithm/control subsystem/steering switch/rear steering switch ==
  RR 2w : Inport
  LR 2w : Inport  Port=2
  steering in : Inport  Port=3
  RR 4w : Inport  Port=4
  LR 4w : Inport  Port=5
  Switch : Switch  Criteria=u2 > Threshold  Threshold=1
  Switch1 : Switch  Criteria=u2 > Threshold  Threshold=1
  steering in1 : InportShadow  Port=3
  steering RR : Outport
  steering LR : Outport  Port=2
  wires:
  RR 2w/1 -> Switch/3
  LR 4w/1 -> Switch1/1
  steering in/1 -> Switch/2
  Switch/1 -> steering RR/1
  LR 2w/1 -> Switch1/3
  Switch1/1 -> steering LR/1
  steering in1/1 -> Switch1/2
  RR 4w/1 -> Switch/1

== system HANcoder_E407_SMV_program/HANcoder STM32 Target - E407-STM32 algorithm/control subsystem/steering switch/speed back ==
  LR 2w : Inport
  RR 2w : Inport  Port=2
  steering in : Inport  Port=3
  LR 4w : Inport  Port=4
  RR 4w : Inport  Port=5
  Switch : Switch  Criteria=u2 > Threshold  Threshold=1
  Switch1 : Switch  Criteria=u2 > Threshold  Threshold=1
  steering in1 : InportShadow  Port=3
  speed LR : Outport
  speed RR : Outport  Port=2
  wires:
  steering in1/1 -> Switch1/2
  Switch1/1 -> speed RR/1
  Switch/1 -> speed LR/1
  steering in/1 -> Switch/2
  LR 4w/1 -> Switch/1
  LR 2w/1 -> Switch/3
  RR 4w/1 -> Switch1/1
  RR 2w/1 -> Switch1/3

== system HANcoder_E407_SMV_program/HANcoder STM32 Target - E407-STM32 algorithm/control subsystem/steering switch/speed front ==
  LF 2w : Inport
  RF 2w : Inport  Port=2
  steering in : Inport  Port=3
  LF 4w : Inport  Port=4
  RF 4w : Inport  Port=5
  Switch : Switch  Criteria=u2 > Threshold  Threshold=1
  Switch1 : Switch  Criteria=u2 > Threshold  Threshold=1
  steering in1 : InportShadow  Port=3
  speed LF : Outport
  speed RF : Outport  Port=2
  wires:
  LF 2w/1 -> Switch/3
  RF 4w/1 -> Switch1/1
  steering in/1 -> Switch/2
  Switch/1 -> speed LF/1
  RF 2w/1 -> Switch1/3
  Switch1/1 -> speed RF/1
  steering in1/1 -> Switch1/2
  LF 4w/1 -> Switch/1

== system HANcoder_E407_SMV_program/HANcoder STM32 Target - E407-STM32 algorithm/Xbee controll/Check received data/Check next 3 bytes and send via CAN/Enabled Subsystem ==
  In1 : Inport
  In2 : Inport  Port=2
  Enable : EnablePort
  Out1 : Outport
  Out2 : Outport  Port=2
  wires:
  In1/1 -> Out1/1
  In2/1 -> Out2/1

== system HANcoder_E407_SMV_program/HANcoder STM32 Target - E407-STM32 algorithm/Xbee controll/Check received data/Check next 3 bytes and send via CAN/UART stop ==
  Level-2 M-file S-Function : M-S-Function  FunctionName=sfcn_uart_receive  Parameters=tsamp
  Term1 : Terminator
  Out1 : Outport
  wires:
  Level-2 M-file S-Function/2 -> Term1/1
  Level-2 M-file S-Function/1 -> Out1/1

== system HANcoder_E407_SMV_program/HANcoder STM32 Target - E407-STM32 algorithm/Xbee controll/Check received data/Check next 3 bytes and send via CAN/UART value1 ==
  Level-2 M-file S-Function : M-S-Function  FunctionName=sfcn_uart_receive  Parameters=tsamp
  Term1 : Terminator
  Out1 : Outport
  wires:
  Level-2 M-file S-Function/2 -> Term1/1
  Level-2 M-file S-Function/1 -> Out1/1

== system HANcoder_E407_SMV_program/HANcoder STM32 Target - E407-STM32 algorithm/Xbee controll/Check received data/Check next 3 bytes and send via CAN/UART value2 ==
  Level-2 M-file S-Function : M-S-Function  FunctionName=sfcn_uart_receive  Parameters=tsamp
  Term1 : Terminator
  Out1 : Outport
  wires:
  Level-2 M-file S-Function/1 -> Out1/1
  Level-2 M-file S-Function/2 -> Term1/1

== system HANcoder_E407_SMV_program/HANcoder STM32 Target - E407-STM32 algorithm/Xbee controll/Check received data/Check received data/Check next 3 bytes and send via CAN ==
  note: Here we check the next three bytes, the priority determines which byte is read first from the buffer. Priority can be changed by right clicking the block and selecting properties
  note: This should be replaced by a checksum
  note: Only use the signals when the last byte is valid
  Enable : EnablePort
  Check if it is the stop byte : simulink/Logic and Bit Operations/Compare To Constant  relop===  const=253  OutDataTypeStr=uint8
  Enabled Subsystem : Subsystem  TreatAsAtomicUnit=on
  UART stop : Subsystem  Tag=HANcoder_TARGET_STM32_E407  Priority=30  AncestorBlock=HANcoder_STM32_Target/STM32-E407/UART/UART receive  mask(UART receive){channel=UART1: CON3 - D1 & D0, useStatusOut=off, tsamp=-1}
      mask prompts: useStatusOut "Use status outport"; tsamp "Sample time"
      mask help:
      | Function
      | ==========
      | Reads a byte from the UART reception buffer.
      |
      | Parameters per channel
      | ======================
      | - Select channel (TX & RX)
      | - Select if the status output should be enabled.
      |
      | Outputs
      | =======
      | - The value of the receive byte.
      | - When the status output is 0, the reception buffer was empty.
      mask init:
      | uartChannelInfoStr = sfcn_uart_receive_mcb(2, channel, useStatusOut);
      settings: MoveFcn=drawLogos
      mask Help: web('sfcn_uart_receive.html')
      mask TypeOptions channel: UART1: CON3 - D1 & D0 | UART2: CON PD - 8 & 9 | UART3: CON PD - 11 & 12 | UART6: UEXT - 3 & 4
      mask Display: fprintf('UART receive\n%s', uartChannelInfoStr);patch([240 246 246],[8 14 2],[1 0 0]);patch([248 248 254],[14 2 8],[0 0 0.35]);
  UART value1 : Subsystem  Tag=HANcoder_TARGET_STM32_E407  Priority=10  AncestorBlock=HANcoder_STM32_Target/STM32-E407/UART/UART receive  mask(UART receive){channel=UART1: CON3 - D1 & D0, useStatusOut=off, tsamp=-1}
      mask prompts: useStatusOut "Use status outport"; tsamp "Sample time"
      mask help:
      | Function
      | ==========
      | Reads a byte from the UART reception buffer.
      |
      | Parameters per channel
      | ======================
      | - Select channel (TX & RX)
      | - Select if the status output should be enabled.
      |
      | Outputs
      | =======
      | - The value of the receive byte.
      | - When the status output is 0, the reception buffer was empty.
      mask init:
      | uartChannelInfoStr = sfcn_uart_receive_mcb(2, channel, useStatusOut);
      settings: MoveFcn=drawLogos
      mask Help: web('sfcn_uart_receive.html')
      mask TypeOptions channel: UART1: CON3 - D1 & D0 | UART2: CON PD - 8 & 9 | UART3: CON PD - 11 & 12 | UART6: UEXT - 3 & 4
      mask Display: fprintf('UART receive\n%s', uartChannelInfoStr);patch([240 246 246],[8 14 2],[1 0 0]);patch([248 248 254],[14 2 8],[0 0 0.35]);
  UART value2 : Subsystem  Tag=HANcoder_TARGET_STM32_E407  Priority=20  AncestorBlock=HANcoder_STM32_Target/STM32-E407/UART/UART receive  mask(UART receive){channel=UART1: CON3 - D1 & D0, useStatusOut=off, tsamp=-1}
      mask prompts: useStatusOut "Use status outport"; tsamp "Sample time"
      mask help:
      | Function
      | ==========
      | Reads a byte from the UART reception buffer.
      |
      | Parameters per channel
      | ======================
      | - Select channel (TX & RX)
      | - Select if the status output should be enabled.
      |
      | Outputs
      | =======
      | - The value of the receive byte.
      | - When the status output is 0, the reception buffer was empty.
      mask init:
      | uartChannelInfoStr = sfcn_uart_receive_mcb(2, channel, useStatusOut);
      settings: MoveFcn=drawLogos
      mask Help: web('sfcn_uart_receive.html')
      mask TypeOptions channel: UART1: CON3 - D1 & D0 | UART2: CON PD - 8 & 9 | UART3: CON PD - 11 & 12 | UART6: UEXT - 3 & 4
      mask Display: fprintf('UART receive\n%s', uartChannelInfoStr);patch([240 246 246],[8 14 2],[1 0 0]);patch([248 248 254],[14 2 8],[0 0 0.35]);
  drive_mode : Outport
  steer_mode : Outport  Port=2
  wires:
  Enabled Subsystem/2(Out2) -> steer_mode/1
  Enabled Subsystem/1(Out1) -> drive_mode/1
  UART value2/1(Out1) -> Enabled Subsystem/2(In2)
  UART value1/1(Out1) -> Enabled Subsystem/1(In1)
  Check if it is the stop byte/1 -> Enabled Subsystem/Enable
  UART stop/1(Out1) -> Check if it is the stop byte/1
